simulink model "Baldosas_10"  (R2023b)
settings: Solver=VariableStepAuto  StartTime=0.0  StopTime=10.0  RelTol=1e-3
libraries: arduinosensorlib x2, simulink x1
settings Model: Creator=Diego  LastModifiedBy=Diego

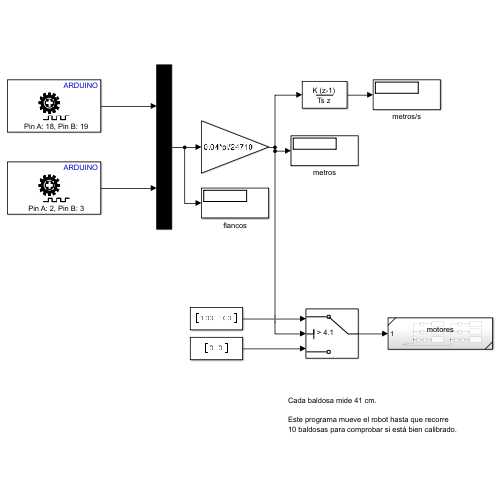
[thumbnail: Simulink's stored preview of the top-level diagram]
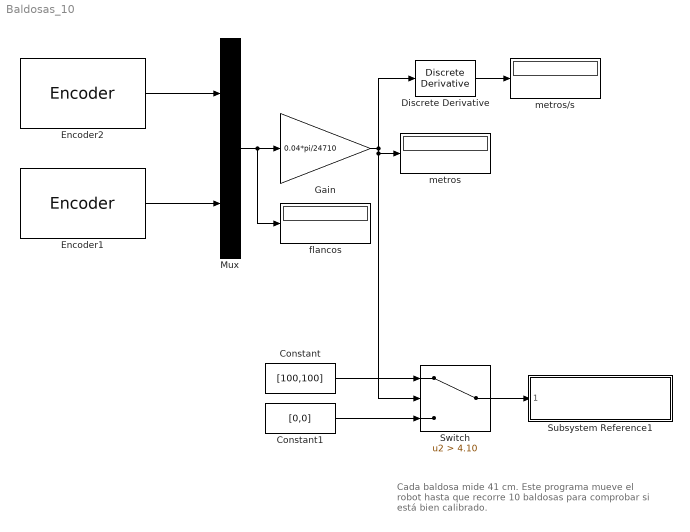
== system Baldosas_10 ==
  note: Cada baldosa mide 41 cm.
      |
      | Este programa mueve el robot hasta que recorre
      | 10 baldosas para comprobar si está bien calibrado.
  Constant : Constant  Value=[100,100]
  Constant1 : Constant  Value=[0,0]
  Discrete Derivative : simulink/Discrete/Discrete Derivative  gainval=1.0  ICPrevScaledInput=0.0  OutMin=[]  OutMax=[]  OutDataType=fixdt(1, 16)  OutScaling=2^-10  DoSatur=off
  Encoder1 : arduinosensorlib/Encoder  InputA=2  InputB=3  Mode=No reset  SampleTime=-1
  Encoder2 : arduinosensorlib/Encoder  InputA=18  InputB=19  Mode=No reset  SampleTime=-1
  Gain : Gain  Gain=0.04*pi/24710
  Mux : Mux  Inputs=2
  Subsystem Reference1 : Subsystem  ReferencedSubsystem=motores
  Switch : Switch  Criteria=u2 > Threshold  Threshold=4.10  SaturateOnIntegerOverflow=off  InputSameDT=off
  flancos : Display
  metros : Display
  metros/s : Display
  wires:
  Discrete Derivative/1 -> metros/s/1
  Gain/1 -> Discrete Derivative/1, Switch/2, metros/1
  Encoder2/1 -> Mux/1
  Encoder1/1 -> Mux/2
  Mux/1 -> flancos/1, Gain/1
  Constant/1 -> Switch/1
  Constant1/1 -> Switch/3
  Switch/1 -> Subsystem Reference1/1
